simulink model "MPPT_ANFIS_testing"  (R2023a)
settings: Solver=ode45  StartTime=0.0  StopTime=1  FixedStep=1e-5  MaxStep=1e-4  RelTol=10e-4  EnableMultiTasking=on
libraries: spsSeriesRLCBranchLib x6, spsStairGeneratorLib x4, spsIdealSwitchLib x3, spsVoltageMeasurementLib x2, fuzblock x1, slpidlib x1, powerlib_extras x1, spsDiodeLib x1, spsGroundLib x1, spsIGBTDiodeLib x1, spsCurrentMeasurementLib x1, spsPVArrayLib x1
settings Model: Creator=Administrator  LastModifiedBy=marga
settings SolverCC: AlgebraicLoopSolver=TrustRegion
settings DataIOCC: LimitDataPoints=on  SaveFormat=Array  SignalLoggingSaveFormat=ModelDataLogs  ReturnWorkspaceOutputs=off
settings OptimizationCC: ExpressionDepthLimit=2147483647  LifeSpan=inf
settings DebuggingCC: UnderspecifiedInitializationDetection=Classic  MergeDetectMultiDrivingBlocksExec=none  SolverPrmCheckMsg=warning  FcnCallInpInsideContextMsg=warning  UnconnectedInputMsg=warning  UnconnectedOutputMsg=warning  UnconnectedLineMsg=warning  StateNameClashWarn=warning  SFUnexpectedBacktrackingDiag=warning  SFNoUnconditionalDefaultTransitionDiag=warning  SFExecutionAtInitializationDiag=none  ArithmeticOperatorsInVariantConditions=warning
settings HardwareCC: ProdBitPerPointer=32  ProdBitPerSizeT=32  ProdBitPerPtrDiffT=32  ProdLargestAtomicFloat=None  ProdIntDivRoundTo=Undefined  ProdEndianess=Unspecified  ProdWordSize=32  ProdHWDeviceType=32-bit Generic
settings ModelReferenceCC: EnableRefExpFcnMdlSchedulingChecks=on  PropagateSignalLabelsOutOfModel=off
settings SFSimCC: SimUseLocalCustomCode=off  CustomCodeUndefinedFunction=UseInterfaceOnly
settings RTWCC: RTWUseLocalCustomCode=off
settings CodeAppCC: StateflowObjectComments=on
settings GRTTargetCC: TargetLangStandard=C89/C90 (ANSI)  CombineOutputUpdateFcns=off  GRTInterface=on
settings ConfigComp: CovMetricSettings=dw  CovSaveCumulativeToWorkspaceVar=on  CovSaveSingleToWorkspaceVar=on  CovExternalEMLEnable=off
settings SimscapeCC: SimscapeNormalizeSystem=off

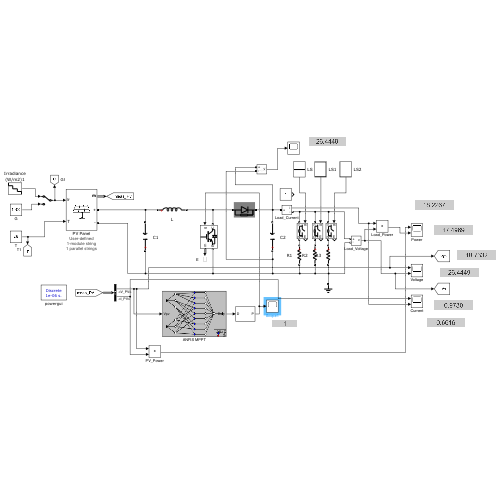
[thumbnail: Simulink's stored preview of the top-level diagram]
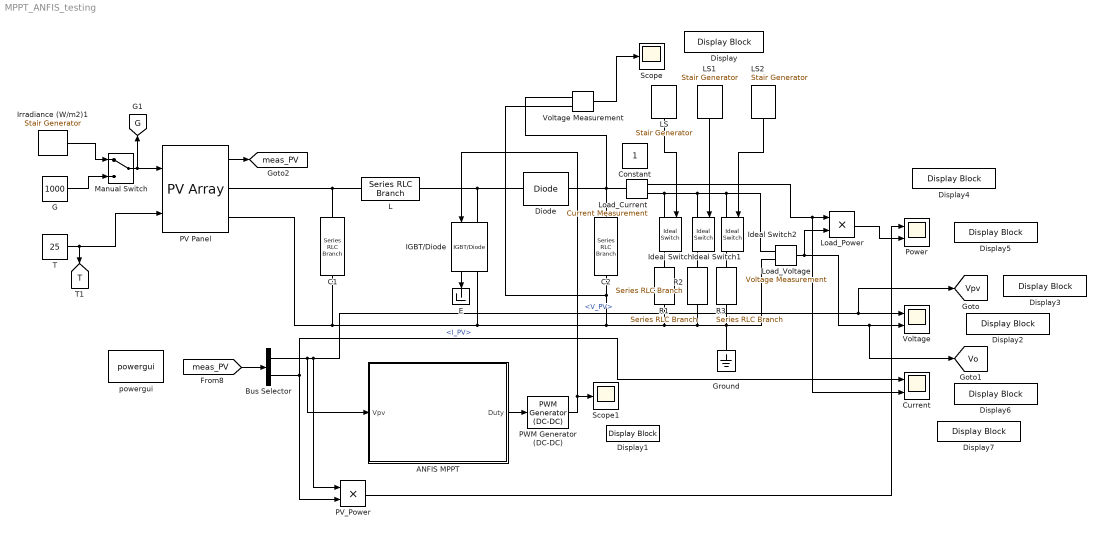
== system MPPT_ANFIS_testing ==
  ANFIS MPPT : Subsystem
      mask Display: image('E:\B.tech\4-1\Project Capstone\3.png'); % Use "Edit Image" on toolstrip to change.
  Bus Selector : BusSelector  OutputSignals=V_PV,I_PV
  C1 : spsSeriesRLCBranchLib/Series RLC Branch  LConnTagsString=__new0  RConnTagsString=__new0  BranchType=C  Resistance=1  Inductance=1e-3  SetiL0=off  InitialCurrent=0  Capacitance=100e-6  Setx0=off  InitialVoltage=0  Measurements=None
  C2 : spsSeriesRLCBranchLib/Series RLC Branch  LConnTagsString=__new0  RConnTagsString=__new0  BranchType=C  Resistance=1  Inductance=1e-3  SetiL0=off  InitialCurrent=0  Capacitance=100e-6  Setx0=off  InitialVoltage=0  Measurements=None
  Constant : Constant
  Current : Scope  NumInputPorts=2
  Diode : spsDiodeLib/Diode  Ron=0.001  Lon=0  Vf=0.8  IC=0  UseSnubber=off  Rs=500  Cs=250e-9  Measurements=off
  Display{,1..7} (8 alike) : DisplayBlock  LabelPosition=Hide  Transparency=1
  E : Terminator
  G : Constant  Value=1000
  Ground : spsGroundLib/Ground  LConnTagsString=a
  IGBT/Diode : spsIGBTDiodeLib/IGBT//Diode  Ron=1e-3  Rs=1e5  Cs=inf  Measurements=on
  Ideal Switch : spsIdealSwitchLib/Ideal Switch  Ron=0.001  Lon=0  IC=0  Rs=1e5  Cs=inf  Measurements=on
  Ideal Switch1 : spsIdealSwitchLib/Ideal Switch  Ron=0.001  Lon=0  IC=0  Rs=1e5  Cs=inf  Measurements=on
  Ideal Switch2 : spsIdealSwitchLib/Ideal Switch  Ron=0.001  Lon=0  IC=0  Rs=1e5  Cs=inf  Measurements=on
  Irradiance (W/m2)1 : spsStairGeneratorLib/Stair Generator  t=[0, 0.2 , 0.4 , 0.6, 0.8]  e=[1,0.8,0.6,0.4, 0.2]*1000  Ts=0.0001
  L : spsSeriesRLCBranchLib/Series RLC Branch  LConnTagsString=__new0  RConnTagsString=__new0  BranchType=L  Resistance=1  Inductance=3e-3  SetiL0=off  InitialCurrent=0  Capacitance=1e-6  Setx0=off  InitialVoltage=0  Measurements=None
  LS : spsStairGeneratorLib/Stair Generator  t=[0, 0.3]  e=[1, 0]  Ts=0.0001
  LS1 : spsStairGeneratorLib/Stair Generator  t=[0, 0.3, 0.6]  e=[0, 1, 0]  Ts=0.0001
  LS2 : spsStairGeneratorLib/Stair Generator  t=[0, 0.3, 0.6]  e=[0, 0, 1]  Ts=0.0001
  Load_Current : spsCurrentMeasurementLib/Current Measurement  PhasorSimulation=off  OutputType=Complex  PSBequivalent=0
  Load_Power : Product  RndMeth=Zero
  Load_Voltage : spsVoltageMeasurementLib/Voltage Measurement  PhasorSimulation=off  OutputType=Complex  PSBequivalent=0
  Manual Switch : ManualSwitch
  PV Panel : spsPVArrayLib/PV Array  Npar=1  Nser=1  PlotType=one module @ 25 deg.C & specified irradiances  S_vec="[ 1000 800  600  400 200 100 50]"  Temp_C_vec="[ 45 25  ]"  ModuleName=User-defined  PlotWhenSelected=off  Pm=99.912  Ncell=36  Voc=22.2  Isc=5.76  Vm=18.4  Im=5.43  beta_Voc_pc=-0.36901  alpha_Isc_pc=0.086998  beta_Voc=-0.08192  alpha_Isc=0.0050111  IL=5.7902  I0=2.7663e-10  nI=1.0107  Rsh=232.6069  Rs=0.18596  RobustModel=off  RobustCellTemperature=313.3991  BAL=off  Tc=1e-6  Tfilter=1e-5
      settings: AttributesFormatString=|
      | %<ModuleName>
      | %<Nser>-module string
      | %<Npar> parallel strings
  PV_Power : Product  RndMeth=Zero
  PWM Generator (DC-DC) : spsPWMGeneratorDCDCLib/PWM Generator (DC-DC)  Fsw=10000  Ts=0
  Power : Scope  NumInputPorts=2
  R1 : spsSeriesRLCBranchLib/Series RLC Branch  LConnTagsString=__new0  RConnTagsString=__new0  BranchType=R  Resistance=20  Inductance=1e-3  SetiL0=off  InitialCurrent=0  Capacitance=1e-6  Setx0=off  InitialVoltage=0  Measurements=None
  R2 : spsSeriesRLCBranchLib/Series RLC Branch  LConnTagsString=__new0  RConnTagsString=__new0  BranchType=R  Resistance=30  Inductance=1e-3  SetiL0=off  InitialCurrent=0  Capacitance=1e-6  Setx0=off  InitialVoltage=0  Measurements=None
  R3 : spsSeriesRLCBranchLib/Series RLC Branch  LConnTagsString=__new0  RConnTagsString=__new0  BranchType=R  Resistance=40  Inductance=1e-3  SetiL0=off  InitialCurrent=0  Capacitance=1e-6  Setx0=off  InitialVoltage=0  Measurements=None
  Scope : Scope
  Scope1 : Scope
  T : Constant  Value=25
  Voltage : Scope  NumInputPorts=2
  Voltage Measurement : spsVoltageMeasurementLib/Voltage Measurement  PhasorSimulation=off  OutputType=Complex  PSBequivalent=0
  powergui : sps_lib/powergui  Priority=1  SimulationMode=Discrete  SampleTime=1e-6  frequency=60  Iterations=50  frequencyindice=0  Pbase=100e6  ErrMax=1e-4  UnitsV=kV  UnitsW=MW  buscounter=0  FunctionMessages=off  echomessages=off  EnableUseOfTLC=off  CurrentSourceSwitches=off  DisableSnubberDevices=off  DisableRonSwitches=off  DisableVfSwitches=off  DisplayEquations=off  AutomaticDiscreteSolvers=off  SolverType=Tustin/Backward Euler (TBE)  Interpol=off  ExternalGateDelay=off  methode=off  Ts=100  x0status=blocks  SPID=on  SwTol=0  HookPort=off  NonlinearTolerance=1e-4  nMaxIteration=100  ContinueOnMaxIteration=off  RestoreLinks=warning  ResistiveCurrentMeasurement=off  Frange=[0:2:500]  Ylog=off  Xlog=on  ShowGrid=off  save=off  variable=ZData  structure=0  ZoomFFT=off  StartTime=0.0  cycles=1  DisplayStyle=1  fundamental=60  FreqAxis=off  MaxFrequency=1000  frequencyindicesteady=1  RmsSteady=1  display=off
  tag scope: G=global, T=global, Vo=global, Vpv=global, meas_PV=global
  wires:
  T/1 -> [T], PV Panel/2
  IGBT/Diode/1 -> E/1
  PV Panel/1 -> [meas_PV]
  [meas_PV] -> Bus Selector/1
  Bus Selector/2 -> Current/1, PV_Power/2  "<I_PV>"
  Bus Selector/1 -> [Vpv], Voltage/1, PV_Power/1, ANFIS MPPT/1(Vpv)  "<V_PV>"
  Load_Voltage/1 -> [Vo], Voltage/2, Load_Power/2
  Load_Current/1 -> Current/2, Load_Power/1
  Load_Power/1 -> Power/2
  PV_Power/1 -> Power/1
  Manual Switch/1 -> PV Panel/1, [G]
  Irradiance (W/m2)1/1 -> Manual Switch/1
  G/1 -> Manual Switch/2
  PWM Generator (DC-DC)/1 -> Scope1/1, IGBT/Diode/1
  ANFIS MPPT/1(Duty) -> PWM Generator (DC-DC)/1
  LS/1 -> Ideal Switch/1
  LS1/1 -> Ideal Switch1/1
  LS2/1 -> Ideal Switch2/1
  Voltage Measurement/1 -> Scope/1
  connections:
  L/LConn1 -- PV Panel/RConn1 -- C1/RConn1
  L/RConn1 -- Diode/LConn1 -- IGBT/Diode/LConn1
  R2/RConn1 -- Ground/LConn1 -- Load_Voltage/LConn2 -- R3/RConn1 -- R1/RConn1 -- Voltage Measurement/LConn2 -- C2/LConn1 -- PV Panel/RConn2 -- C1/LConn1 -- IGBT/Diode/RConn1
  Diode/RConn1 -- C2/RConn1 -- Voltage Measurement/LConn1 -- Load_Current/LConn1
  Load_Current/RConn1 -- Ideal Switch2/LConn1 -- Load_Voltage/LConn1 -- Ideal Switch1/LConn1 -- Ideal Switch/LConn1
  Ideal Switch/RConn1 -- R1/LConn1
  Ideal Switch1/RConn1 -- R2/LConn1
  Ideal Switch2/RConn1 -- R3/LConn1

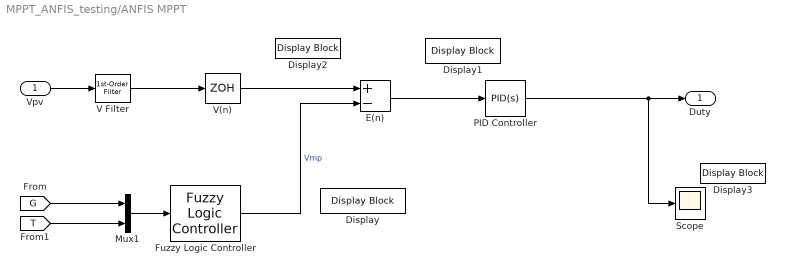
== system MPPT_ANFIS_testing/ANFIS MPPT ==
  Vpv : Inport
  Display{,1..3} (4 alike) : DisplayBlock  LabelPosition=Hide  Transparency=1
  E(n) : Sum  Inputs=+-
  Fuzzy Logic Controller : fuzblock/Fuzzy Logic  Controller  FIS='labpaneldata.fis'  OutputSampleNumber=101  DataType=double  FuzzifiedInputs=off  RuleFiringStrengths=off  RuleOutputs=off  AggregatedOutputs=off  SimulateUsing=Interpreted execution  OutOfRangeInputValueMessage=warning  NoRuleFiredMessage=warning  EmptyOutputFuzzySetMessage=warning
  Mux1 : Mux  Inputs=2
  PID Controller : slpidlib/PID Controller  Controller=PID  Form=Parallel  TimeDomain=Continuous-time  UseExternalTs=off  SampleTime=-1  IntegratorMethod=Forward Euler  FilterMethod=Forward Euler  ControllerParametersSource=internal  P=0.6  I=0.3  UseKiTs=off  D=0  N=100  UseFilter=on  TunerSelectOption=Transfer Function Based (PID Tuner App)  InitialConditionSource=internal  InitialConditionForIntegrator=0  InitialConditionForFilter=0  DifferentiatorICPrevScaledInput=0  ExternalReset=none  TrackingMode=off  Kt=1  LimitOutput=off  SatLimitsSource=internal  UpperSaturationLimit=1  LowerSaturationLimit=0  LinearizeAsGain=on  AntiWindupMode=none  Kb=1  LimitIntegrator=off  UpperIntegratorSaturationLimit=inf  LowerIntegratorSaturationLimit=-inf  POutMin=[]  POutMax=[]  IOutMin=[]  IOutMax=[]  DOutMin=[]  DOutMax=[]  NOutMin=[]  NOutMax=[]  SumOutMin=[]  SumOutMax=[]  SaturationOutMin=[]  SaturationOutMax=[]  PParamMin=[]  PParamMax=[]  IParamMin=[]  IParamMax=[]  DParamMin=[]  DParamMax=[]  NParamMin=[]  NParamMax=[]  KbParamMin=[]  KbParamMax=[]  KtParamMin=[]  KtParamMax=[]  KbOutMin=[]  KbOutMax=[]  KtOutMin=[]  KtOutMax=[]  IntegratorOutMin=[]  IntegratorOutMax=[]  FilterOutMin=[]  FilterOutMax=[]  SumI1OutMin=[]  SumI1OutMax=[]  SumI2OutMin=[]  SumI2OutMax=[]  SumI3OutMin=[]  SumI3OutMax=[]  SumI4OutMin=[]  SumI4OutMax=[]  SumDOutMin=[]  SumDOutMax=[]  DifferentiatorOutMin=[]  DifferentiatorOutMax=[]  FilterDiffOutCoefMin=[]  FilterDiffOutCoefMax=[]  ReciprocalOutMin=[]  ReciprocalOutMax=[]  SumDenOutMin=[]  SumDenOutMax=[]  SumNumOutMin=[]  SumNumOutMax=[]  DivideOutMin=[]  DivideOutMax=[]  UdiffTsProdOutMin=[]  UdiffTsProdOutMax=[]  NTsProdOutMin=[]  NTsProdOutMax=[]  UintegralTsProdOutMin=[]  UintegralTsProdOutMax=[]  UngainTsProdOutMin=[]  UngainTsProdOutMax=[]  ClampingZeroOutDataTypeStr=Inherit: Inherit via back propagation  ClampingZeroOutMin=[]  ClampingZeroOutMax=[]  FilterDenConstantOutDataTypeStr=Inherit: Inherit via back propagation  FilterDenConstantOutMin=[]  FilterDenConstantOutMax=[]  PCopyOutDataTypeStr=Inherit: Inherit via back propagation  PCopyOutMin=[]  PCopyOutMax=[]  NCopyOutDataTypeStr=Inherit: Inherit via back propagation  NCopyOutMin=[]  NCopyOutMax=[]  IntegratorContinuousStateAttributes=''  IntegratorStateMustResolveToSignalObject=off  IntegratorRTWStateStorageClass=Auto  FilterContinuousStateAttributes=''  FilterStateMustResolveToSignalObject=off  FilterRTWStateStorageClass=Auto  ParallelPVariant=InternalParameters  IdealPVariant=Disabled  IVariant=InternalParameters  DVariant=InternalParameters  IntegratorVariant=Continuous  SatVariant=Disabled  AWVariant=Passthrough  PCopyVariant=Disabled  TRVariant=Disabled  FdbkBlocksVariant=Forward  IdealPFdbkVariant=Disabled  SatFdbkVariant=Disabled  DerivativeFilterVariant=ContFilter  NVariant=InternalParameters  NCopyVariant=Disabled  FilterICVariant=InternalICsFilter  IntegratorICVariant=InternalICs  ExternalResetVariant=Disabled  TRSumVariant=Passthrough  SumFdbkVariant=Disabled  SumVariant=Sum_PID  TsampFilterVariant=InternalTs  TsampNgainVariant=Passthrough  TsampIntegralVariant=Disabled_SignalSpec  ExternalSaturationOutDataTypeStr=Inherit: Same as second input
  Scope : Scope
  V Filter : powerlib_extras/Control  Blocks/1st-Order  Filter  FilterType=Lowpass  Tc=30e-3  Initialize=off  Vac_Init=[0.8 -25 60]  Vdc_Init=-0.4  PlotResponse=off  param1=[1 500 1]
  V(n) : ZeroOrderHold  SampleTime=1e-4
  Duty : Outport  VectorParamsAs1DForOutWhenUnconnected=off
  wires:
  Vpv/1 -> V Filter/1
  V Filter/1 -> V(n)/1
  V(n)/1 -> E(n)/1
  Fuzzy Logic Controller/1 -> E(n)/2  "Vmp"
  Mux1/1 -> Fuzzy Logic Controller/1
  [G] -> Mux1/1
  [T] -> Mux1/2
  E(n)/1 -> PID Controller/1
  PID Controller/1 -> Scope/1, Duty/1
